simulink model "MS04_SimModel_Battery_management_system"  (R2023a)
settings: Solver=VariableStepAuto  StartTime=0.0  StopTime=3600.0  FixedStep=0.001  RelTol=1e-3
undefined symbols (not defined in the file or in its folder): Ion, Lithium
libraries: spsBatteryLib x30, spsControlledCurrentSourceLib x3, spspowerguiLib x1
settings Model: Creator=trifonov  LastModifiedBy=trifonov

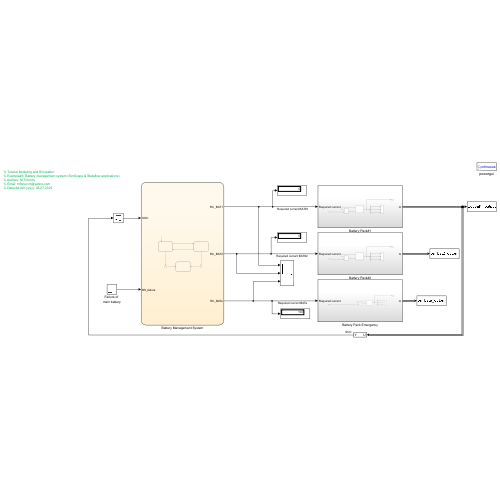
[thumbnail: Simulink's stored preview of the top-level diagram]
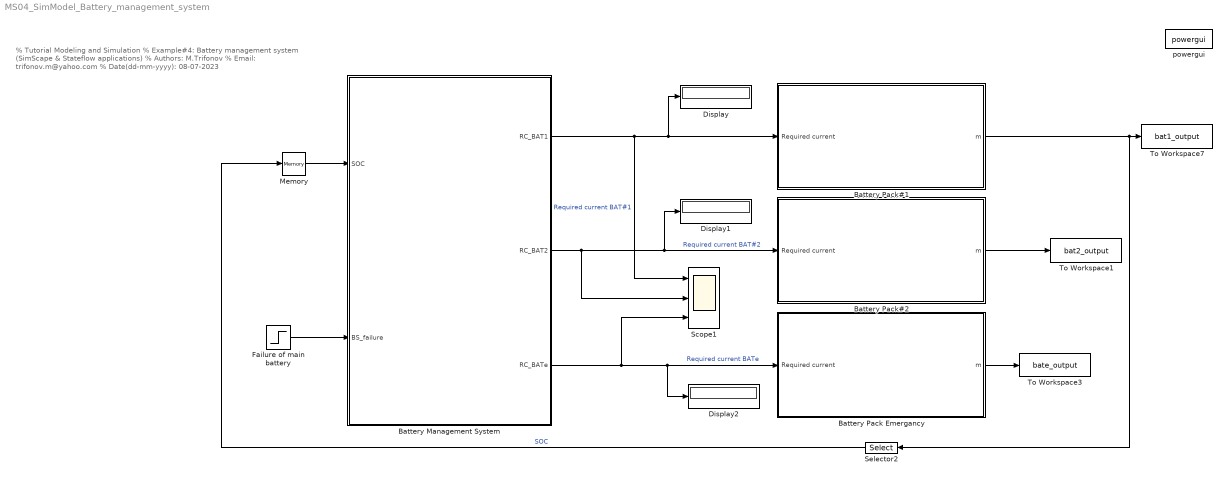
== system MS04_SimModel_Battery_management_system ==
  note: % Tutorial Modeling and Simulation
      | % Example#4: Battery management system (SimScape & Stateflow applications)
      | % Authors: M.Trifonov
      | % Email: trifonov.m@yahoo.com
      | % Date(dd-mm-yyyy): 08-07-2023
  Battery Management System : Stateflow chart  TreatAsAtomicUnit=on
      settings: PortSchema="{\"entries\":[{\"content\":{\"sides\":[{\"content\":{\"connectorIds\":[\"In1\",\"In2\"]},\"type\":\"ConnectorPlacement.EquallySpacedRectSide\",\"uuid\":\"fb8b0fde-b6b7-45bf-9e39-6367451fb1a3\"},{\"content\":{\"connectorIds\":[\"Out2\",\"Out3\",\"Out1\"],\"side\":\"RIGHT\"},\"type\":\"ConnectorPlacement.EquallySpacedRectSide\",\"uuid\":\"d114c820-8c32-4885-8443-446919f40098\"},{\"content\":{\"side\":\"TOP\"},\"type\":\"ConnectorPlacement.EquallySpacedRectSide\",\"uuid\":\"da8117e0-a67b-4275-8434-d0e14033deda\"}]},\"type\":\"ConnectorPlacement.EquallySpacedConnector\",\"uuid\":\"e02754af-b16e-4cd7-8588-844a97499f7d\"}],\"packageUris\":[\"http://schema.mathworks.com/mf0/Connector/R2020b\"],\"version\":\"1.0\"}"
  Battery Pack Emergancy : Subsystem
  Battery Pack#1 : Subsystem
  Battery Pack#2 : Subsystem
  Display : Display
  Display1 : Display
  Display2 : Display
  Failure of main battery : Step  Time=2700  SampleTime=0
  Memory : Memory  InitialCondition=100
  Scope1 : Scope  NumInputPorts=3
  Selector2 : Selector  InputPortWidth=3  IndexOptions=Index vector (dialog)  Indices=1:1  OutputSizes=1
  To Workspace1 : ToWorkspace  VariableName=bat2_output  SampleTime=-1
      settings: Save2DSignal=2-D array (concatenate along first dimension)
  To Workspace3 : ToWorkspace  VariableName=bate_output  SampleTime=-1
      settings: Save2DSignal=2-D array (concatenate along first dimension)
  To Workspace7 : ToWorkspace  VariableName=bat1_output  SampleTime=-1
      settings: Save2DSignal=2-D array (concatenate along first dimension)
  powergui : spspowerguiLib/powergui  SimulationMode=Continuous  SampleTime=1e-6  frequency=60  Iterations=50  frequencyindice=0  Pbase=100e6  ErrMax=1e-4  UnitsV=kV  UnitsW=MW  buscounter=0  FunctionMessages=off  echomessages=off  EnableUseOfTLC=off  CurrentSourceSwitches=off  DisableSnubberDevices=off  DisableRonSwitches=off  DisableVfSwitches=off  DisplayEquations=off  AutomaticDiscreteSolvers=off  SolverType=Tustin  Interpol=off  ExternalGateDelay=off  methode=off  Ts=0  x0status=blocks  SPID=off  SwTol=0  HookPort=off  NonlinearTolerance=1e-4  nMaxIteration=100  ContinueOnMaxIteration=off  RestoreLinks=warning  ResistiveCurrentMeasurement=off  Frange=[0:2:500]  Ylog=off  Xlog=on  ShowGrid=off  save=off  variable=ZData  structure=0  ZoomFFT=on  StartTime=0.0  cycles=1  DisplayStyle=1  fundamental=60  FreqAxis=off  MaxFrequency=1000  frequencyindicesteady=1  RmsSteady=1  display=off
  wires:
  Battery Pack#1/1(m) -> Selector2/1, To Workspace7/1
  Battery Management System/2(RC_BAT1) -> Scope1/1, Battery Pack#1/1(Required current), Display/1  "Required current BAT#1"
  Battery Pack#2/1(m) -> To Workspace1/1
  Battery Management System/3(RC_BAT2) -> Scope1/2, Display1/1, Battery Pack#2/1(Required current)  "Required current BAT#2"
  Selector2/1 -> Memory/1  "SOC"
  Memory/1 -> Battery Management System/1(SOC)
  Battery Management System/1(RC_BATe) -> Scope1/3, Battery Pack Emergancy/1(Required current), Display2/1  "Required current BATe"
  Battery Pack Emergancy/1(m) -> To Workspace3/1
  Failure of main battery/1 -> Battery Management System/2(BS_failure)

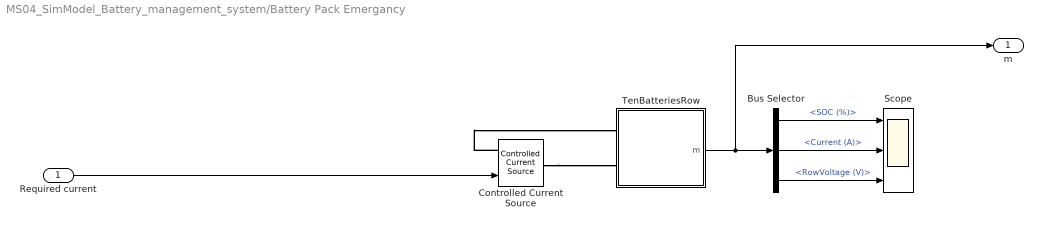
== system MS04_SimModel_Battery_management_system/Battery Pack Emergancy ==
  Required current : Inport
  Bus Selector : BusSelector  OutputSignals=SOC (%),Current (A),RowVoltage (V)
  Controlled Current Source : spsControlledCurrentSourceLib/Controlled Current Source  Initialize=on  Source_Type=AC  Amplitude=0  Phase=0  Frequency=0  Measurements=None
  Scope : Scope  NumInputPorts=3
  TenBatteriesRow : Subsystem
  m : Outport
  wires:
  Required current/1 -> Controlled Current Source/1
  Bus Selector/3 -> Scope/3  "<RowVoltage (V)>"
  Bus Selector/1 -> Scope/1  "<SOC (%)>"
  Bus Selector/2 -> Scope/2  "<Current (A)>"
  TenBatteriesRow/1(m) -> Bus Selector/1, m/1
  connections:
  Controlled Current Source/RConn1 -- TenBatteriesRow/LConn2
  Controlled Current Source/LConn1 -- TenBatteriesRow/LConn1

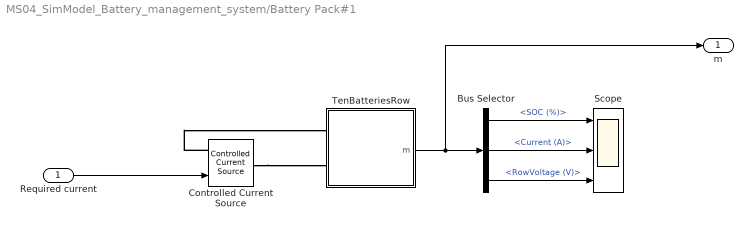
== system MS04_SimModel_Battery_management_system/Battery Pack#1 ==
  Required current : Inport
  Bus Selector : BusSelector  OutputSignals=SOC (%),Current (A),RowVoltage (V)
  Controlled Current Source : spsControlledCurrentSourceLib/Controlled Current Source  Initialize=on  Source_Type=AC  Amplitude=0  Phase=0  Frequency=0  Measurements=None
  Scope : Scope  NumInputPorts=3
  TenBatteriesRow : Subsystem
  m : Outport
  wires:
  Required current/1 -> Controlled Current Source/1
  Bus Selector/3 -> Scope/3  "<RowVoltage (V)>"
  Bus Selector/1 -> Scope/1  "<SOC (%)>"
  Bus Selector/2 -> Scope/2  "<Current (A)>"
  TenBatteriesRow/1(m) -> Bus Selector/1, m/1
  connections:
  Controlled Current Source/RConn1 -- TenBatteriesRow/LConn2
  Controlled Current Source/LConn1 -- TenBatteriesRow/LConn1

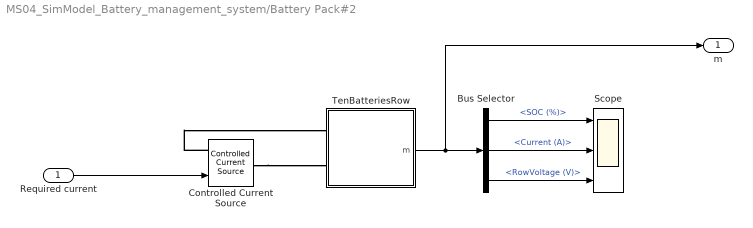
== system MS04_SimModel_Battery_management_system/Battery Pack#2 ==
  Required current : Inport
  Bus Selector : BusSelector  OutputSignals=SOC (%),Current (A),RowVoltage (V)
  Controlled Current Source : spsControlledCurrentSourceLib/Controlled Current Source  Initialize=on  Source_Type=AC  Amplitude=0  Phase=0  Frequency=0  Measurements=None
  Scope : Scope  NumInputPorts=3
  TenBatteriesRow : Subsystem
  m : Outport
  wires:
  TenBatteriesRow/1(m) -> m/1, Bus Selector/1
  Bus Selector/2 -> Scope/2  "<Current (A)>"
  Bus Selector/1 -> Scope/1  "<SOC (%)>"
  Bus Selector/3 -> Scope/3  "<RowVoltage (V)>"
  Required current/1 -> Controlled Current Source/1
  connections:
  Controlled Current Source/LConn1 -- TenBatteriesRow/LConn1
  Controlled Current Source/RConn1 -- TenBatteriesRow/LConn2

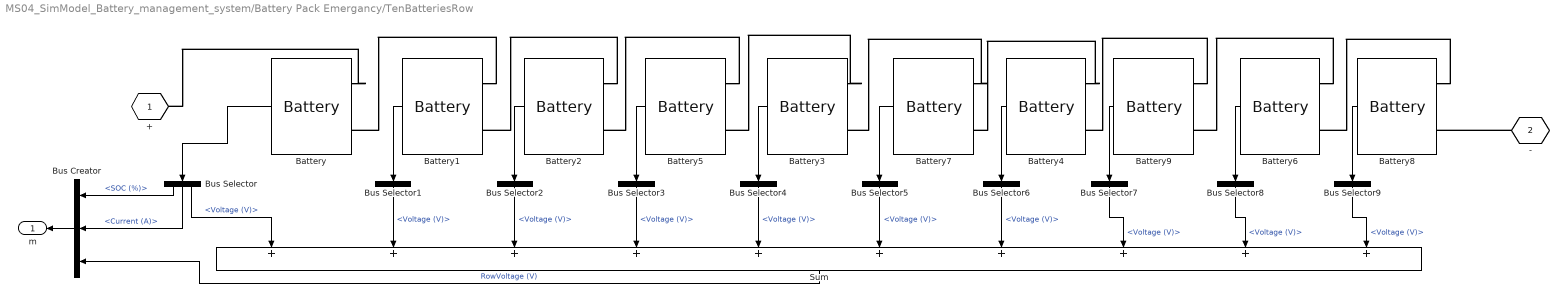
== system MS04_SimModel_Battery_management_system/Battery Pack Emergancy/TenBatteriesRow ==
  Battery{,1..9} (10 alike) : spsBatteryLib/Battery  BatType=Lithium-Ion  ShowTempParam=off  ThermalPreset=no  ShowAgeParam=off  NomV=3.7  NomQ=41  SOC=100  Batt_Tr=30  PresetModel=off  MaxQ=45  MinV=2.7  FullV=4.2  Dis_rate=320  R=0.013333  Normal_OP=7  expZone="[4      0.2653]"  current=[6.5 13 32.5]  Units=Time  Tci=20  NomT=20  T2=-30  MaxQ2=4.8  FullV2=7.1  Normal_OP2=5.655  expZone2="[6.58           1]"  Rca=0.6  ti=2000  Dp=0  Neq0=0  Tsim=1e6  Ta1=25  Qeol=5.4*0.9  Reol=0.013333*1.2  Char_age=[2.3478, 3]  Dis_age=[2.3478, 10]  N1=1500  N2=10500  N3=1000  N4=1400  Ta2=45  N5=950
      settings: LibrarySourceBlock=electricdrivelib/Extra Sources/Battery
  Bus Creator : BusCreator  Inputs=3
  Bus Selector : BusSelector  OutputSignals=SOC (%),Current (A),Voltage (V)
  Bus Selector{1..9} (9 alike) : BusSelector  OutputSignals=Voltage (V)
  Sum : Sum  Inputs=++++++++++
  "+ " : PMIOPort  Tag=PMCPort  Side=Left
  - : PMIOPort  Tag=PMCPort  Port=2  Side=Left
  m : Outport  VectorParamsAs1DForOutWhenUnconnected=off
  wires:
  Bus Selector/1 -> Bus Creator/1  "<SOC (%)>"
  Sum/1 -> Bus Creator/3  "RowVoltage (V)"
  Bus Selector9/1 -> Sum/10  "<Voltage (V)>"
  Bus Selector8/1 -> Sum/9  "<Voltage (V)>"
  Bus Selector7/1 -> Sum/8  "<Voltage (V)>"
  Bus Selector6/1 -> Sum/7  "<Voltage (V)>"
  Bus Selector5/1 -> Sum/6  "<Voltage (V)>"
  Bus Selector4/1 -> Sum/5  "<Voltage (V)>"
  Bus Selector3/1 -> Sum/4  "<Voltage (V)>"
  Bus Selector2/1 -> Sum/3  "<Voltage (V)>"
  Bus Selector1/1 -> Sum/2  "<Voltage (V)>"
  Battery8/1 -> Bus Selector9/1
  Battery6/1 -> Bus Selector8/1
  Battery9/1 -> Bus Selector7/1
  Battery4/1 -> Bus Selector6/1
  Battery7/1 -> Bus Selector5/1
  Battery3/1 -> Bus Selector4/1
  Battery5/1 -> Bus Selector3/1
  Battery2/1 -> Bus Selector2/1
  Battery1/1 -> Bus Selector1/1
  Bus Creator/1 -> m/1
  Bus Selector/3 -> Sum/1  "<Voltage (V)>"
  Bus Selector/2 -> Bus Creator/2  "<Current (A)>"
  Battery/1 -> Bus Selector/1
  connections:
  Battery4/LConn1 -- Battery7/LConn2
  Battery7/LConn1 -- Battery3/LConn2
  Battery9/LConn1 -- Battery4/LConn2
  Battery5/LConn1 -- Battery2/LConn2
  Battery/LConn1 -- "+ "/RConn1
  Battery6/LConn1 -- Battery9/LConn2
  Battery1/LConn1 -- Battery/LConn2
  Battery8/LConn1 -- Battery6/LConn2
  -/RConn1 -- Battery8/LConn2
  Battery3/LConn1 -- Battery5/LConn2
  Battery2/LConn1 -- Battery1/LConn2

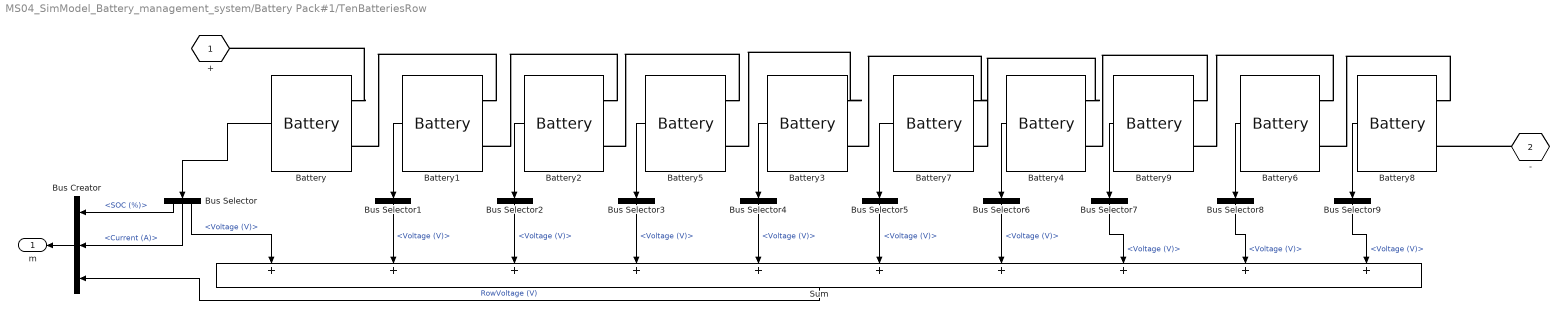
== system MS04_SimModel_Battery_management_system/Battery Pack#1/TenBatteriesRow ==
  Battery{,1..9} (10 alike) : spsBatteryLib/Battery  BatType=Lithium-Ion  ShowTempParam=off  ThermalPreset=no  ShowAgeParam=off  NomV=3.7  NomQ=41  SOC=100  Batt_Tr=30  PresetModel=off  MaxQ=45  MinV=2.7  FullV=4.2  Dis_rate=320  R=0.013333  Normal_OP=7  expZone="[4      0.2653]"  current=[6.5 13 32.5]  Units=Time  Tci=20  NomT=20  T2=-30  MaxQ2=4.8  FullV2=7.1  Normal_OP2=5.655  expZone2="[6.58           1]"  Rca=0.6  ti=2000  Dp=0  Neq0=0  Tsim=1e6  Ta1=25  Qeol=5.4*0.9  Reol=0.013333*1.2  Char_age=[2.3478, 3]  Dis_age=[2.3478, 10]  N1=1500  N2=10500  N3=1000  N4=1400  Ta2=45  N5=950
      settings: LibrarySourceBlock=electricdrivelib/Extra Sources/Battery
  Bus Creator : BusCreator  Inputs=3
  Bus Selector : BusSelector  OutputSignals=SOC (%),Current (A),Voltage (V)
  Bus Selector{1..9} (9 alike) : BusSelector  OutputSignals=Voltage (V)
  Sum : Sum  Inputs=++++++++++
  "+ " : PMIOPort  Tag=PMCPort  Side=Left
  - : PMIOPort  Tag=PMCPort  Port=2  Side=Left
  m : Outport  VectorParamsAs1DForOutWhenUnconnected=off
  wires:
  Bus Selector/1 -> Bus Creator/1  "<SOC (%)>"
  Sum/1 -> Bus Creator/3  "RowVoltage (V)"
  Bus Selector9/1 -> Sum/10  "<Voltage (V)>"
  Bus Selector8/1 -> Sum/9  "<Voltage (V)>"
  Bus Selector7/1 -> Sum/8  "<Voltage (V)>"
  Bus Selector6/1 -> Sum/7  "<Voltage (V)>"
  Bus Selector5/1 -> Sum/6  "<Voltage (V)>"
  Bus Selector4/1 -> Sum/5  "<Voltage (V)>"
  Bus Selector3/1 -> Sum/4  "<Voltage (V)>"
  Bus Selector2/1 -> Sum/3  "<Voltage (V)>"
  Bus Selector1/1 -> Sum/2  "<Voltage (V)>"
  Battery8/1 -> Bus Selector9/1
  Battery6/1 -> Bus Selector8/1
  Battery9/1 -> Bus Selector7/1
  Battery4/1 -> Bus Selector6/1
  Battery7/1 -> Bus Selector5/1
  Battery3/1 -> Bus Selector4/1
  Battery5/1 -> Bus Selector3/1
  Battery2/1 -> Bus Selector2/1
  Battery1/1 -> Bus Selector1/1
  Bus Creator/1 -> m/1
  Bus Selector/3 -> Sum/1  "<Voltage (V)>"
  Bus Selector/2 -> Bus Creator/2  "<Current (A)>"
  Battery/1 -> Bus Selector/1
  connections:
  Battery4/LConn1 -- Battery7/LConn2
  Battery7/LConn1 -- Battery3/LConn2
  Battery9/LConn1 -- Battery4/LConn2
  Battery5/LConn1 -- Battery2/LConn2
  Battery/LConn1 -- "+ "/RConn1
  Battery6/LConn1 -- Battery9/LConn2
  Battery1/LConn1 -- Battery/LConn2
  Battery8/LConn1 -- Battery6/LConn2
  -/RConn1 -- Battery8/LConn2
  Battery3/LConn1 -- Battery5/LConn2
  Battery2/LConn1 -- Battery1/LConn2

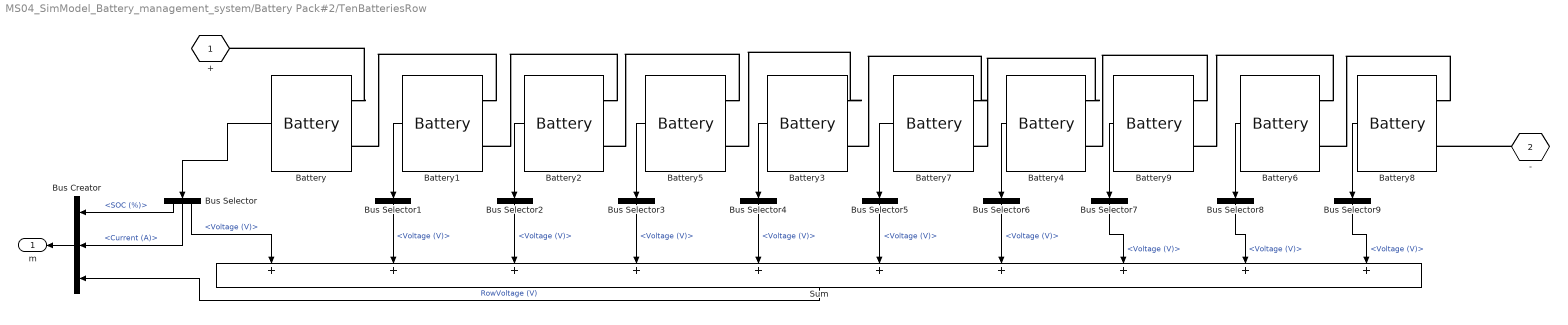
== system MS04_SimModel_Battery_management_system/Battery Pack#2/TenBatteriesRow ==
  Battery{,1..9} (10 alike) : spsBatteryLib/Battery  BatType=Lithium-Ion  ShowTempParam=off  ThermalPreset=no  ShowAgeParam=off  NomV=3.7  NomQ=41  SOC=100  Batt_Tr=30  PresetModel=off  MaxQ=45  MinV=2.7  FullV=4.2  Dis_rate=320  R=0.013333  Normal_OP=7  expZone="[4      0.2653]"  current=[6.5 13 32.5]  Units=Time  Tci=20  NomT=20  T2=-30  MaxQ2=4.8  FullV2=7.1  Normal_OP2=5.655  expZone2="[6.58           1]"  Rca=0.6  ti=2000  Dp=0  Neq0=0  Tsim=1e6  Ta1=25  Qeol=5.4*0.9  Reol=0.013333*1.2  Char_age=[2.3478, 3]  Dis_age=[2.3478, 10]  N1=1500  N2=10500  N3=1000  N4=1400  Ta2=45  N5=950
      settings: LibrarySourceBlock=electricdrivelib/Extra Sources/Battery
  Bus Creator : BusCreator  Inputs=3
  Bus Selector : BusSelector  OutputSignals=SOC (%),Current (A),Voltage (V)
  Bus Selector{1..9} (9 alike) : BusSelector  OutputSignals=Voltage (V)
  Sum : Sum  Inputs=++++++++++
  "+ " : PMIOPort  Tag=PMCPort  Side=Left
  - : PMIOPort  Tag=PMCPort  Port=2  Side=Left
  m : Outport  VectorParamsAs1DForOutWhenUnconnected=off
  wires:
  Battery/1 -> Bus Selector/1
  Bus Selector/2 -> Bus Creator/2  "<Current (A)>"
  Bus Selector/3 -> Sum/1  "<Voltage (V)>"
  Bus Creator/1 -> m/1
  Battery1/1 -> Bus Selector1/1
  Battery2/1 -> Bus Selector2/1
  Battery5/1 -> Bus Selector3/1
  Battery3/1 -> Bus Selector4/1
  Battery7/1 -> Bus Selector5/1
  Battery4/1 -> Bus Selector6/1
  Battery9/1 -> Bus Selector7/1
  Battery6/1 -> Bus Selector8/1
  Battery8/1 -> Bus Selector9/1
  Bus Selector1/1 -> Sum/2  "<Voltage (V)>"
  Bus Selector2/1 -> Sum/3  "<Voltage (V)>"
  Bus Selector3/1 -> Sum/4  "<Voltage (V)>"
  Bus Selector4/1 -> Sum/5  "<Voltage (V)>"
  Bus Selector5/1 -> Sum/6  "<Voltage (V)>"
  Bus Selector6/1 -> Sum/7  "<Voltage (V)>"
  Bus Selector7/1 -> Sum/8  "<Voltage (V)>"
  Bus Selector8/1 -> Sum/9  "<Voltage (V)>"
  Bus Selector9/1 -> Sum/10  "<Voltage (V)>"
  Sum/1 -> Bus Creator/3  "RowVoltage (V)"
  Bus Selector/1 -> Bus Creator/1  "<SOC (%)>"
  connections:
  Battery2/LConn1 -- Battery1/LConn2
  Battery3/LConn1 -- Battery5/LConn2
  -/RConn1 -- Battery8/LConn2
  Battery8/LConn1 -- Battery6/LConn2
  Battery1/LConn1 -- Battery/LConn2
  Battery6/LConn1 -- Battery9/LConn2
  Battery/LConn1 -- "+ "/RConn1
  Battery5/LConn1 -- Battery2/LConn2
  Battery9/LConn1 -- Battery4/LConn2
  Battery7/LConn1 -- Battery3/LConn2
  Battery4/LConn1 -- Battery7/LConn2

== stateflow chart MS04_SimModel_Battery_management_system/Battery Management System ==
  state On
    RC_BAT1=60;
    RC_BAT2=40;
    RC_BATe=0;
  state Off
    RC_BAT1=20;
    RC_BAT2=80;
    RC_BATe=0;
  state Off1
    RC_BAT1=0;
    RC_BAT2=0;
    RC_BATe=100;
  (default) -> On
  On -> Off [order 1] : [SOC<=40]
  Off -> On [order 1] : [SOC>40]
  On -> (junction 18) [order 2] : [BS_failure==1]
  Off -> (junction 22) [order 2] : [BS_failure==1]
  (junction 18) -> Off1
  (junction 22) -> Off1
  data: SOC input; RC_BATe output; RC_BAT1 output; RC_BAT2 output; BS_failure input
